simulink model "stanley"  (R2023b)
settings: Solver=VariableStepAuto  StartTime=0.0  StopTime=150  RelTol=1e-3
StopFcn:
  | % save sstr_4.71_1_2_2.mat
  | % save pstr_4.71_1_2_2_0.95_10.mat
  | % save su_4.71_19_1_1.mat
  | save pu_4.71_19_1_1_0.98_25.mat
model workspace (MAT data in the model file):
  Nc = 4
  Np = 10
libraries: simulink x2, Solver_SF x1
settings Model: Creator=Lenovo  LastModifiedBy=Lenovo
settings SolverCC: AlgebraicLoopSolver=TrustRegion
settings DataIOCC: ReturnWorkspaceOutputs=off
settings DebuggingCC: UnconnectedInputMsg=warning  UnconnectedOutputMsg=warning  UnconnectedLineMsg=warning  ArithmeticOperatorsInVariantConditions=warning
settings ModelReferenceCC: EnableRefExpFcnMdlSchedulingChecks=on
settings SFSimCC: SimUseLocalCustomCode=off  CustomCodeUndefinedFunction=UseInterfaceOnly
settings RTWCC: RTWUseLocalCustomCode=off

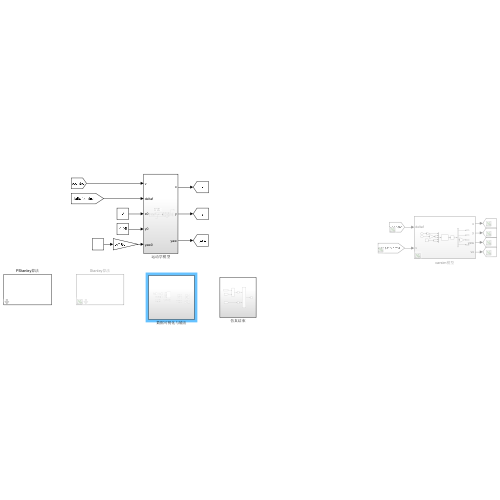
[thumbnail: Simulink's stored preview of the top-level diagram]
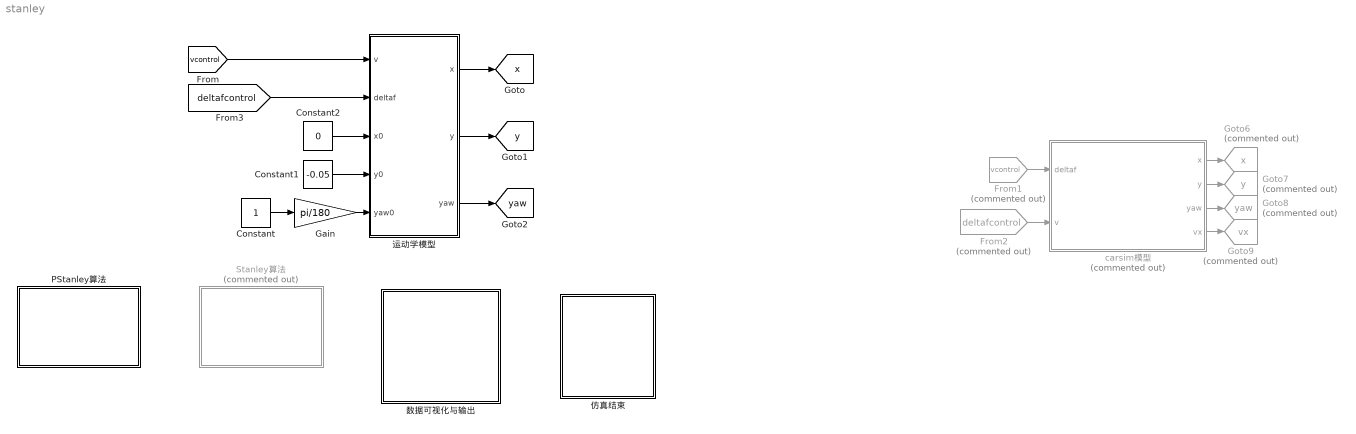
== system stanley ==
  Constant : Constant
  Constant1 : Constant  Value=-0.05
  Constant2 : Constant  Value=0
  From1 : From  Commented=on  GotoTag=vcontrol  TagVisibility=global
  From2 : From  Commented=on  GotoTag=deltafcontrol  TagVisibility=global
  Gain : Gain  Gain=pi/180
  Goto6 : Goto  Commented=on  GotoTag=x  TagVisibility=global
  Goto7 : Goto  Commented=on  GotoTag=y  TagVisibility=global
  Goto8 : Goto  Commented=on  GotoTag=yaw  TagVisibility=global
  Goto9 : Goto  Commented=on  GotoTag=vx  TagVisibility=global
  PStanley算法 : Subsystem  mask{k_y=19, k_v=1, c=1, k0=0.98, Np=25}
      mask DialogControl ParameterGroupVar Prompt: 参数
  Stanley算法 : Subsystem  Commented=on  mask{k_y=19, k_v=1, c=1}
      mask DialogControl ParameterGroupVar Prompt: 参数
  carsim模型 : Subsystem  Commented=on
  仿真结束 : Subsystem
  数据可视化与输出 : Subsystem
  运动学模型 : Subsystem
  tag scope: x=global, y=global, yaw=global
  wires:
  carsim模型/1(x) -> Goto6/1
  carsim模型/2(y) -> Goto7/1
  carsim模型/3(yaw) -> Goto8/1
  carsim模型/4(vx) -> Goto9/1
  From2/1 -> carsim模型/2(v)
  From1/1 -> carsim模型/1(deltaf)
  运动学模型/2(y) -> [y]
  Constant/1 -> Gain/1
  Constant2/1 -> 运动学模型/3(x0)
  运动学模型/3(yaw) -> [yaw]
  [vcontrol] -> 运动学模型/1(v)
  Gain/1 -> 运动学模型/5(yaw0)
  Constant1/1 -> 运动学模型/4(y0)
  [deltafcontrol] -> 运动学模型/2(deltaf)
  运动学模型/1(x) -> [x]

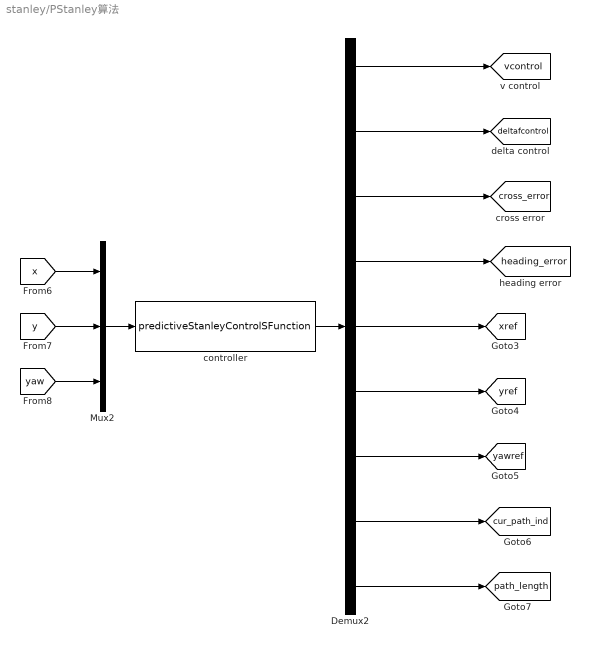
== system stanley/PStanley算法 ==
  Demux2 : Demux  Outputs=9
  Mux2 : Mux  Inputs=3
  controller : S-Function  FunctionName=predictiveStanleyControlSFunction  Parameters=k_y, k_v, c, k0, Np  SFunctionDeploymentMode=off  EnableBusSupport=off
  tag scope: cross_error=global, cur_path_ind=global, deltafcontrol=global, heading_error=global, path_length=global, vcontrol=global, xref=global, yawref=global, yref=global
  wires:
  Demux2/5 -> [xref]
  Demux2/4 -> [heading_error]
  [yaw] -> Mux2/3
  Demux2/8 -> [cur_path_ind]
  Demux2/6 -> [yref]
  Demux2/9 -> [path_length]
  Demux2/3 -> [cross_error]
  Demux2/2 -> [deltafcontrol]
  [y] -> Mux2/2
  [x] -> Mux2/1
  Demux2/1 -> [vcontrol]
  Mux2/1 -> controller/1
  Demux2/7 -> [yawref]
  controller/1 -> Demux2/1

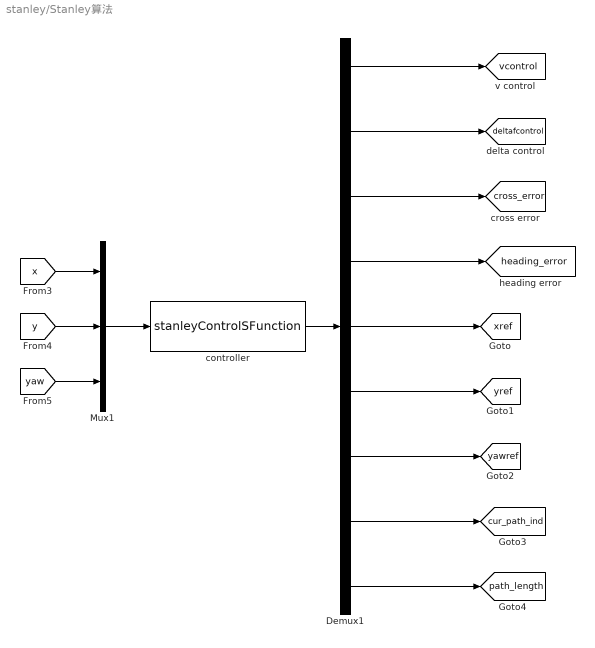
== system stanley/Stanley算法 ==
  Demux1 : Demux  Outputs=9
  Mux1 : Mux  Inputs=3
  controller : S-Function  FunctionName=stanleyControlSFunction  Parameters=k_y, k_v, c  SFunctionDeploymentMode=off  EnableBusSupport=off
  tag scope: cross_error=global, cur_path_ind=global, deltafcontrol=global, heading_error=global, path_length=global, vcontrol=global, xref=global, yawref=global, yref=global
  wires:
  Demux1/3 -> [cross_error]
  Demux1/1 -> [vcontrol]
  Demux1/2 -> [deltafcontrol]
  Mux1/1 -> controller/1
  [y] -> Mux1/2
  Demux1/4 -> [heading_error]
  [x] -> Mux1/1
  controller/1 -> Demux1/1
  [yaw] -> Mux1/3
  Demux1/5 -> [xref]
  Demux1/6 -> [yref]
  Demux1/7 -> [yawref]
  Demux1/8 -> [cur_path_ind]
  Demux1/9 -> [path_length]

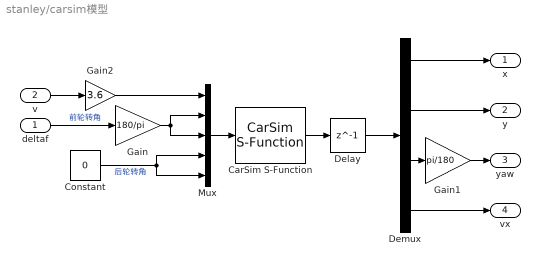
== system stanley/carsim模型 ==
  deltaf : Inport
  v : Inport  Port=2
  CarSim S-Function : Solver_SF/CarSim S-Function  Priority=1  SIMFILE=simfile.sim  Run_RTs=off  vs_state_ind=Run  StopMode_ind=Vehicle Model
  Constant : Constant  Value=0
  Delay : Delay  DelayLength=1
  Demux : Demux
  Gain : Gain  Gain=180/pi
  Gain1 : Gain  Gain=pi/180
  Gain2 : Gain  Gain=3.6
  Mux : Mux  Inputs=5
  x : Outport  VectorParamsAs1DForOutWhenUnconnected=off
  y : Outport  Port=2  VectorParamsAs1DForOutWhenUnconnected=off
  yaw : Outport  Port=3  VectorParamsAs1DForOutWhenUnconnected=off
  vx : Outport  Port=4  VectorParamsAs1DForOutWhenUnconnected=off
  wires:
  Mux/1 -> CarSim S-Function/1
  CarSim S-Function/1 -> Delay/1
  Demux/1 -> x/1
  Demux/2 -> y/1
  Demux/3 -> Gain1/1
  Gain1/1 -> yaw/1
  Demux/4 -> vx/1
  Delay/1 -> Demux/1
  Gain2/1 -> Mux/1
  v/1 -> Gain2/1
  Gain/1 -> Mux/2, Mux/3
  Constant/1 -> Mux/5, Mux/4  "后轮转角"
  deltaf/1 -> Gain/1  "前轮转角"

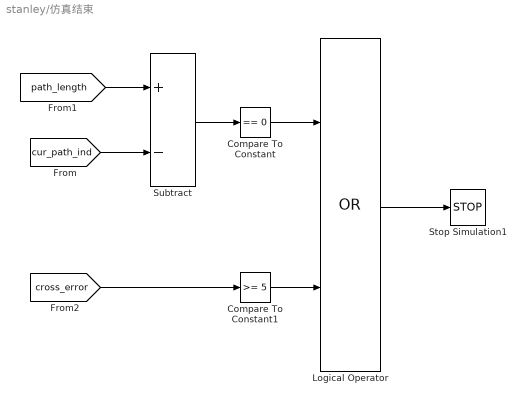
== system stanley/仿真结束 ==
  Compare To Constant : simulink/Logic and Bit Operations/Compare To Constant  relop===  const=0  OutDataTypeStr=boolean
  Compare To Constant1 : simulink/Logic and Bit Operations/Compare To Constant  relop=>=  const=5  OutDataTypeStr=boolean
  Logical Operator : Logic  Operator=OR  AllPortsSameDT=off  OutDataTypeStr=boolean
  Stop Simulation1 : Stop
  Subtract : Sum  Inputs=+-
  wires:
  [path_length] -> Subtract/1
  [cur_path_ind] -> Subtract/2
  Subtract/1 -> Compare To Constant/1
  [cross_error] -> Compare To Constant1/1
  Compare To Constant1/1 -> Logical Operator/2
  Compare To Constant/1 -> Logical Operator/1
  Logical Operator/1 -> Stop Simulation1/1

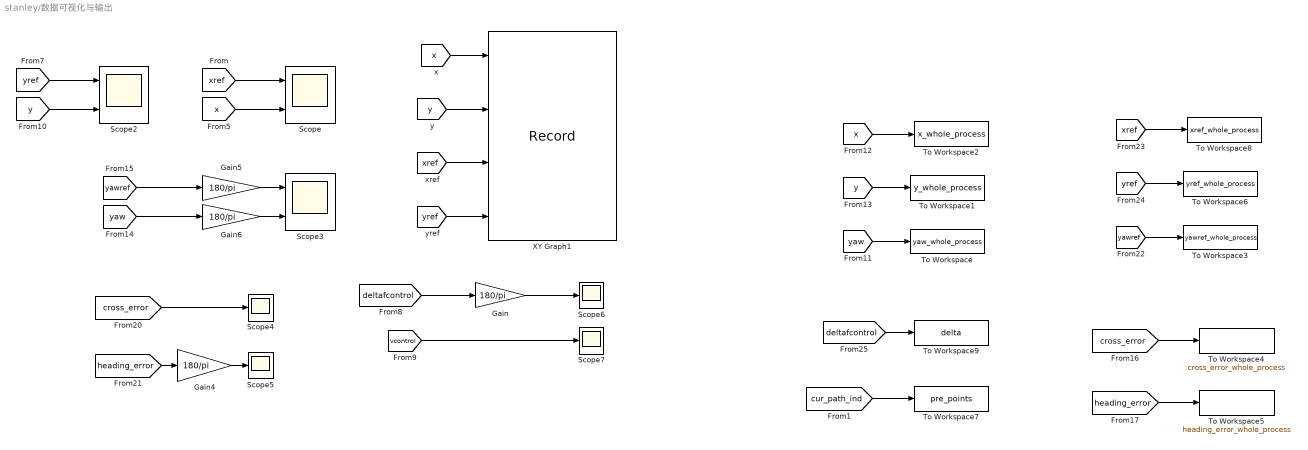
== system stanley/数据可视化与输出 ==
  Gain{,4..6} (4 alike) : Gain  Gain=180/pi
  Scope : Scope  NumInputPorts=2
  Scope2 : Scope  NumInputPorts=2
  Scope3 : Scope  NumInputPorts=2
  Scope{4..7} (4 alike) : Scope
  To Workspace : ToWorkspace  VariableName=yaw_whole_process  SampleTime=0.1
  To Workspace1 : ToWorkspace  VariableName=y_whole_process  SampleTime=0.1
      settings: Save2DSignal=2-D array (concatenate along first dimension)
  To Workspace2 : ToWorkspace  VariableName=x_whole_process  SampleTime=0.1
      settings: Save2DSignal=2-D array (concatenate along first dimension)
  To Workspace3 : ToWorkspace  VariableName=yawref_whole_process  SampleTime=0.1
  To Workspace4 : ToWorkspace  VariableName=cross_error_whole_process  SampleTime=0.1
      settings: Save2DSignal=2-D array (concatenate along first dimension)
  To Workspace5 : ToWorkspace  VariableName=heading_error_whole_process  SampleTime=0.1
      settings: Save2DSignal=2-D array (concatenate along first dimension)
  To Workspace6 : ToWorkspace  VariableName=yref_whole_process  SampleTime=0.1
      settings: Save2DSignal=2-D array (concatenate along first dimension)
  To Workspace7 : ToWorkspace  VariableName=pre_points  SampleTime=0.1
      settings: Save2DSignal=2-D array (concatenate along first dimension)
  To Workspace8 : ToWorkspace  VariableName=xref_whole_process  SampleTime=0.1
      settings: Save2DSignal=2-D array (concatenate along first dimension)
  To Workspace9 : ToWorkspace  VariableName=delta  SampleTime=0.1
      settings: Save2DSignal=2-D array (concatenate along first dimension)
  XY Graph1 : Record  FileSettingsInternal="{\"entries\":[{\"content\":{\"excelSettings\":{\"content\":{},\"type\":\"Streamout.ExcelSettings\"}},\"type\":\"Streamout.FileSettingStorage\",\"uuid\":\"\"}],\"packageUris\":[\"http:\\/\\/schema.mathworks.com\\/mf0\\/streamout_blocks\\/R2020a\"],\"version\":\"1.0\"}"  Layout=[1 1]  SignalsInternal="{\"entries\":[{\"content\":{\"signals\":[{\"content\":{\"blockPath\":[],\"dimensions\":[1],\"domain\":\"\",\"lineColor\":\"#64d413\",\"plots\":[1],\"port\":1,\"sid\":[\"\"],\"signalID\":1596,\"signalName\":\"x\"},\"type\":\"RecordBlkView.Signal\",\"uuid\":\"\"},{\"content\":{\"blockPath\":[],\"dimensions\":[1],\"domain\":\"\",\"lineColor\":\"#ff13a6\",\"plots\":[1],\"port\":2,\"sid\":[\"\"],\"signalID\":1600,\"signalName\":\"y\"},\"type\":\"RecordBlkView.Signal\",\"uuid\":\"\"},{\"content\":{\"blockPath\":[],\"dimensions\":[1],\"domain\":\"\",\"lineColor\":\"#fe330a\",\"plots\":[1],\"port\":3,\"sid\":[\"\"],\"signalID\":1604,\"signalName\":\"xref\"},\"type\":\"RecordBlkView.Signal\",\"uuid\":\"\"},{\"content\":{\"blockPath\":[],\"dimensions\":[1],\"domain\":\"\",\"lineColor\":\"#22b573\",\"plots\":[1],\"port\":4,\"sid\":[\"\"],\"signalID\":1608,\"signalName\":\"yref\"},\"type\":\"RecordBlkView.Signal\",\"uuid\":\"\"}]},\"type\":\"RecordBlkView.InputSignals\",\"uuid\":\"\"}],\"packageUris\":[\"http:\\/\\/schema.mathworks.com\\/mf0\\/streamout_blocks\\/R2020a\"],\"version\":\"1.0\"}"  VisualizationBindings="{\"xyplotplugin\":{\"info\":[{\"series\":[{\"bindingParametersList\":[{\"parameter\":\"X-Axis\",\"signalID\":1604,\"signalName\":\"xref\"},{\"parameter\":\"Y-Axis\",\"signalID\":1608,\"signalName\":\"yref\"}],\"seriesID\":42332},{\"bindingParametersList\":[{\"parameter\":\"X-Axis\",\"signalID\":1596,\"signalName\":\"x\"},{\"parameter\":\"Y-Axis\",\"signalID\":1600,\"signalName\":\"y\"}],\"seriesID\":24589}],\"subplotID\":1}]}}"  CompatibilityTag=XY  st=-1
  wires:
  [vcontrol] -> Scope7/1
  [deltafcontrol] -> Gain/1
  [x] -> XY Graph1/1
  Gain/1 -> Scope6/1
  [y] -> XY Graph1/2
  [yaw] -> To Workspace/1
  [y] -> To Workspace1/1
  [x] -> To Workspace2/1
  [cross_error] -> To Workspace4/1
  [heading_error] -> To Workspace5/1
  [xref] -> Scope/1
  [x] -> Scope/2
  [y] -> Scope2/2
  [yref] -> Scope2/1
  [yaw] -> Gain6/1
  [cross_error] -> Scope4/1
  [heading_error] -> Gain4/1
  [yref] -> To Workspace6/1
  [yawref] -> To Workspace3/1
  [xref] -> To Workspace8/1
  Gain4/1 -> Scope5/1
  Gain5/1 -> Scope3/1
  Gain6/1 -> Scope3/2
  [yawref] -> Gain5/1
  [deltafcontrol] -> To Workspace9/1
  [xref] -> XY Graph1/3
  [yref] -> XY Graph1/4
  [cur_path_ind] -> To Workspace7/1

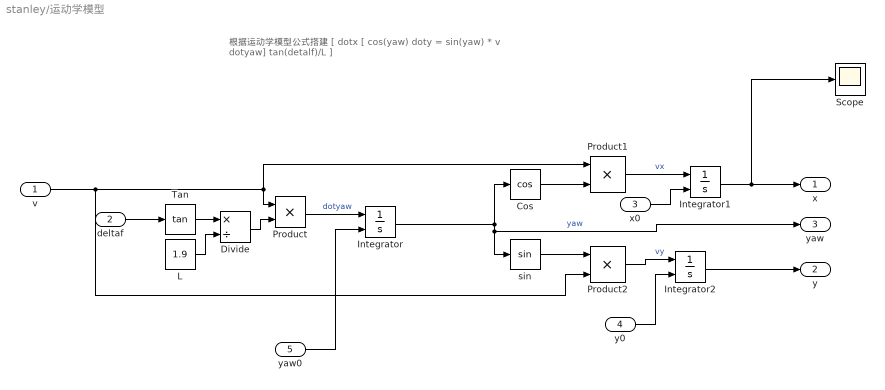
== system stanley/运动学模型 ==
  note: 根据运动学模型公式搭建
      | [ dotx [ cos(yaw)
      | doty = sin(yaw) * v
      | dotyaw] tan(detalf)/L ]
  v : Inport
  deltaf : Inport  Port=2
  x0 : Inport  Port=3
  y0 : Inport  Port=4
  yaw0 : Inport  Port=5
  Cos : Trigonometry  Operator=cos
  Divide : Product  Inputs=*/
  Integrator : Integrator  InitialConditionSource=external
  Integrator1 : Integrator  InitialConditionSource=external
  Integrator2 : Integrator  InitialConditionSource=external
  L : Constant  Value=1.9
  Product : Product
  Product1 : Product
  Product2 : Product
  Scope : Scope
  Tan : Trigonometry  Operator=tan
  sin : Trigonometry
  x : Outport  VectorParamsAs1DForOutWhenUnconnected=off
  y : Outport  Port=2  VectorParamsAs1DForOutWhenUnconnected=off
  yaw : Outport  Port=3  VectorParamsAs1DForOutWhenUnconnected=off
  wires:
  Integrator1/1 -> x/1, Scope/1
  v/1 -> Product/1, Product1/1, Product2/2
  x0/1 -> Integrator1/2
  L/1 -> Divide/2
  y0/1 -> Integrator2/2
  Integrator/1 -> yaw/1, sin/1, Cos/1  "yaw"
  Product1/1 -> Integrator1/1  "vx"
  Product/1 -> Integrator/1  "dotyaw"
  Tan/1 -> Divide/1
  sin/1 -> Product2/1
  Divide/1 -> Product/2
  Integrator2/1 -> y/1
  deltaf/1 -> Tan/1
  Product2/1 -> Integrator2/1  "vy"
  Cos/1 -> Product1/2
  yaw0/1 -> Integrator/2
